simulink model "mpc_modelo"  (R2025a)
settings: Solver=VariableStepAuto  StartTime=0.0  StopTime=10.0  RelTol=1e-3
libraries: mpclib x1
settings Model: Creator=joaof  LastModifiedBy=joaof

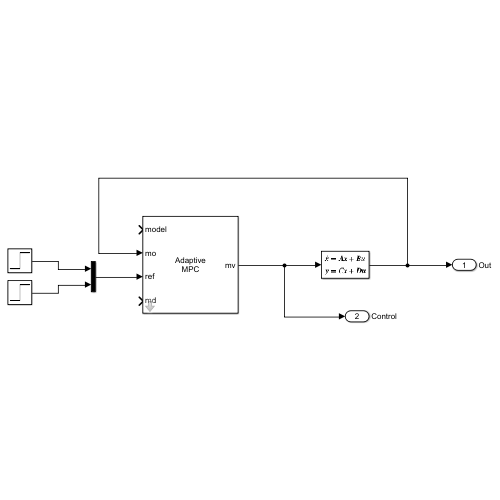
[thumbnail: Simulink's stored preview of the top-level diagram]
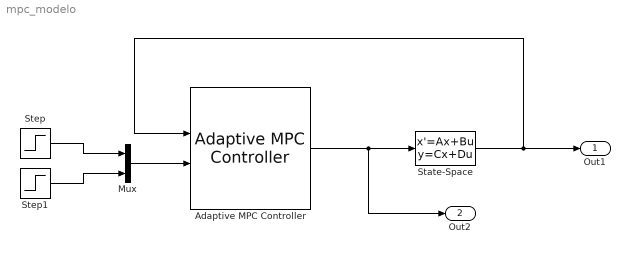
== system mpc_modelo ==
  Adaptive MPC Controller : mpclib/Adaptive MPC Controller  SCDEnableBlockLinearizationSpecification=on  enable_value=0  updateMPCinCallerWorkspace=on  md_inport=on  mv_inport=off  uref_inport=off  return_cost=off  return_mvseq=off  return_qpstatus=off  return_xseq=off  return_state=off  return_ovseq=off  state_inport=off  isltv_plant=off  umin_inport=off  umax_inport=off  ymin_inport=off  ymax_inport=off  cc_inport=off  ywt_inport=off  uwt_inport=off  duwt_inport=off  rhoeps_inport=off  pm_inport=off  MaximumP=10  HorizonChoice=FixedHorizon  BlockDataType=double  SampleTimeInherited=off  switch_inport=off
  Mux : Mux  Inputs=2
  State-Space : StateSpace  InitialCondition=0
  Step : Step  SampleTime=0
  Step1 : Step  SampleTime=0
  Out1 : Outport  SignalName=Out
  Out2 : Outport  Port=2  SignalName=Control
  wires:
  Adaptive MPC Controller/1 -> Out2/1, State-Space/1
  State-Space/1 -> Adaptive MPC Controller/2, Out1/1
  Mux/1 -> Adaptive MPC Controller/3
  Step/1 -> Mux/1
  Step1/1 -> Mux/2
